simulink model "findClosetPt_tgtPt_SlipAngle_th"  (R2020a)
settings: Solver=VariableStepAuto  StartTime=0.0  StopTime=0  RelTol=1e-3
values from neighbouring files (symbols this model uses):
  G_vK = 10*[0;1;1]    [testSilvaCtrl.m]
  kiteLoc = kiteLoc./norm(kiteLoc)    [findIntersectionPoint.m]    (also in testSilvaCtrl.m = cIn.eqPathCoordinates(cIn.aBooth,cIn.bBooth,     cIn.meanEle)
  startPt = 1*0.75*2*pi    (= 4.71238898038)    [testSilvaCtrl.m]
libraries: findClosetPt_tgtPt_SlipAngle x1
settings Model: Creator=Ayaz  LastModifiedBy=Ayaz

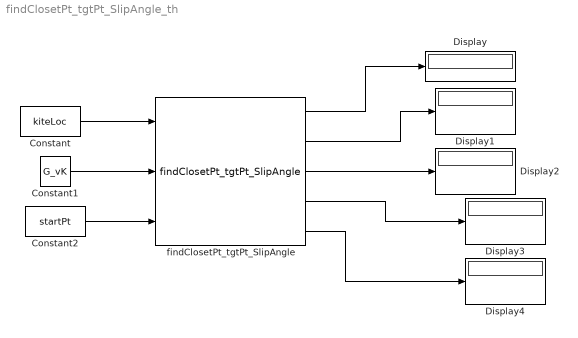
== system findClosetPt_tgtPt_SlipAngle_th ==
  Constant : Constant  Value=kiteLoc
  Constant1 : Constant  Value=G_vK
  Constant2 : Constant  Value=startPt
  Display{,1..4} (5 alike) : Display
  findClosetPt_tgtPt_SlipAngle : findClosetPt_tgtPt_SlipAngle/findClosetPt_tgtPt_SlipAngle  PW=60  PH=28  PE=30  L1=0.05
  wires:
  Constant/1 -> findClosetPt_tgtPt_SlipAngle/1
  Constant1/1 -> findClosetPt_tgtPt_SlipAngle/2
  Constant2/1 -> findClosetPt_tgtPt_SlipAngle/3
  findClosetPt_tgtPt_SlipAngle/1 -> Display/1
  findClosetPt_tgtPt_SlipAngle/2 -> Display1/1
  findClosetPt_tgtPt_SlipAngle/3 -> Display2/1
  findClosetPt_tgtPt_SlipAngle/4 -> Display3/1
  findClosetPt_tgtPt_SlipAngle/5 -> Display4/1
